simulink model "LandingGearMode"  (R2015a)
settings: Solver=FixedStepDiscrete  StartTime=0.0  StopTime=10.0  FixedStep=0.2  RelTol=1e-3
PreLoadFcn:
  | load busdata;
settings Model: RecordCoverage=on  Creator=syoon  LastModifiedBy=syoon
settings OptimizationCC: BlockReduction=off  InlineParams=on  UseDivisionForNetSlopeComputation=on  ExpressionDepthLimit=2147483647  EfficientFloat2IntCast=on  EfficientMapNaN2IntZero=off  OptimizeModelRefInitCode=on  MaxStackSize=inf
settings DebuggingCC: SignalInfNanChecking=error  SignalRangeChecking=error  ReadBeforeWriteMsg=EnableAllAsError  WriteAfterWriteMsg=EnableAllAsError  WriteAfterReadMsg=EnableAllAsError  AlgebraicLoopMsg=error  ArtificialAlgebraicLoopMsg=error  SaveWithDisabledLinksMsg=error  SaveWithParameterizedLinksMsg=error  BlockPriorityViolationMsg=error  SolverPrmCheckMsg=error  InheritedTsInSrcMsg=error  DiscreteInheritContinuousMsg=error  SigSpecEnsureSampleTimeMsg=error  CheckMatrixSingularityMsg=error  IntegerOverflowMsg=error  ParameterUnderflowMsg=error  ParameterPrecisionLossMsg=error  ParameterTunabilityLossMsg=error  UnderSpecifiedDataTypeMsg=error  UnnecessaryDatatypeConvMsg=warning  VectorMatrixConversionMsg=error  SignalLabelMismatchMsg=error  UnconnectedInputMsg=error  UnconnectedOutputMsg=error  UnconnectedLineMsg=error  SFcnCompatibilityMsg=error  BusObjectLabelMismatch=error  RootOutportRequireBusObject=error  ModelReferenceIOMsg=error  ModelReferenceIOMismatchMessage=error  UnknownTsInhSupMsg=error  ModelReferenceDataLoggingMessage=error  StateNameClashWarn=warning  StrictBusMsg=ErrorOnBusTreatedAsVector  NonBusSignalsTreatedAsBus=error  SFUnexpectedBacktrackingDiag=error  SFInvalidInputDataAccessInChartInitDiag=error  SFNoUnconditionalDefaultTransitionDiag=error  SFTransitionOutsideNaturalParentDiag=error  SFUnconditionalTransitionShadowingDiag=error  SFUndirectedBroadcastEventsDiag=error  SFTransitionActionBeforeConditionDiag=error  IntegerSaturationMsg=error
settings HardwareCC: ProdIntDivRoundTo=Zero  ProdEndianess=LittleEndian  ProdHWDeviceType=Intel->x86/Pentium  TargetBitPerLong=64  TargetBitPerPointer=64  TargetIntDivRoundTo=Zero  TargetEndianess=LittleEndian  TargetWordSize=64  TargetHWDeviceType=Intel->x86-64
settings RTWCC: SystemTargetFile=ert.tlc  TemplateMakefile=ert_default_tmf  Description=Embedded Coder  GenerateReport=on  IncludeHyperlinkInReport=on  LaunchReport=on  PortableWordSizes=on  CodeExecutionProfiling=on  CodeProfilingInstrumentation=on  GenerateTraceInfo=on  GenerateTraceReport=on  GenerateTraceReportSl=on  GenerateTraceReportSf=on  GenerateTraceReportEml=on  GenerateCodeMetricsReport=on
settings CodeAppCC: ForceParamTrailComments=on  IgnoreCustomStorageClasses=off  MangleLength=4  CustomSymbolStrType=$N$R$M  ReqsInCode=on
settings ERTTargetCC: UtilityFuncGeneration=Shared location  ParMdlRefBuildCompliant=on  CompOptLevelCompliant=on  ConcurrentExecutionCompliant=on  IncludeMdlTerminateFcn=off  GeneratePreprocessorConditionals=Disable all  SuppressErrorStatus=on  ERTFirstTimeCompliant=on  SupportAbsoluteTime=off  SupportNonFinite=off  SupportComplex=off  SupportContinuousTime=off  SupportVariableSizeSignals=off  ParenthesesLevel=Maximum  ModelStepFunctionPrototypeControlCompliant=on  CPPClassGenCompliant=on  GenerateSharedConstants=off  ERTCustomFileTemplate=example_file_process.tlc  PreserveExpressionOrder=on  PreserveIfCondition=on  EnableSignedLeftShifts=off
settings ConfigComp: Description=Design Verifier Custom Configuration Component  DVModelCoverageObjectives=MCDC  DVMaxTestCaseSteps=500  DVTestSuiteOptimization=CombinedObjectives (Nonlinear Extended)  DVCoverageDataFile=existingcov.cvt  DVDetectActiveLogic=on  DVSaveHarnessModel=on  DVModelReferenceHarness=on  PSVerificationSettings=PrjConfigAndMisra  PSOpenProjectManager=on  PSAutoStubLUT=off

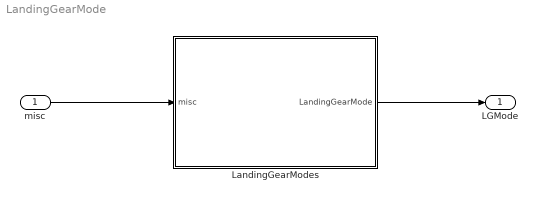
== system LandingGearMode ==
  misc : Inport  RequirementInfo={'other' '..\requirements\DisplaySystemRequirements.docx' '@Simulink_requirement_item_33' 'true' 'The state of the landing gear will be contained in a bus object: MiscData. This bus object is defined as follows:' '' } %GIDa_09af1f37_fea8_4fc2_b25f_3c32d9062372  OutDataTypeStr=Bus: MiscData  PortDimensions=1  SampleTime=0.2  BusOutputAsStruct=on
  LandingGearModes : Stateflow chart  RequirementInfo={'other' '..\requirements\DisplaySystemRequirements.docx' '@Simulink_requirement_item_35' 'true' 'The LGLeftLock and LGRightLock elements of the bus will be used to determine the output of the system: LandingGearMode.' '' } %GIDa_9a49dfa8_e211_495d_8d12_c7afe2a8f08f  TreatAsAtomicUnit=on
      settings: RTWSystemCode=Inline
  LGMode : Outport  RequirementInfo={'other' '..\requirements\DisplaySystemRequirements.docx' '@Simulink_requirement_item_34' 'true' 'The output of the system shall be an integer of type double, LandingGearMode.' '' } %GIDa_2f617b6c_313d_4ee6_8d3d_1e307f4a7039
  wires:
  LandingGearModes/1(LandingGearMode) -> LGMode/1
  misc/1 -> LandingGearModes/1(misc)

== stateflow chart LandingGearMode/LandingGearModes ==
  state LeftLock [parallel]
    settings: executionOrder=1
    state Unlocked
    state Locked
    (default) -> (junction 122)
    (junction 122) -> LeftLock.Unlocked [order 2]
    (junction 122) -> LeftLock.Locked [order 1] : [misc.LGLeftLock]
    LeftLock.Locked -> LeftLock.Unlocked : [~misc.LGLeftLock]
    LeftLock.Unlocked -> LeftLock.Locked : [misc.LGLeftLock]
  state RightLock [parallel]
    settings: executionOrder=2
    state Unlocked
    state Locked
    (default) -> (junction 136)
    (junction 136) -> RightLock.Unlocked [order 2]
    (junction 136) -> RightLock.Locked [order 1] : [misc.LGRightLock]
    RightLock.Locked -> RightLock.Unlocked : [~misc.LGRightLock]
    RightLock.Unlocked -> RightLock.Locked : [misc.LGRightLock]
  state WarningModes [parallel]
    settings: executionOrder=3
    state BothLocked
      entry:
      LandingGearMode = 1;
    state BothUnLocked
      entry:
      LandingGearMode = 3;
    state OnlyOneLocked
      entry:
      LandingGearMode = 2;
    (default) -> (junction 102)
    (junction 102) -> BothLocked [order 1] : [in(LeftLock.Locked) &&...
        | in(RightLock.Locked)]
    (junction 102) -> BothUnLocked [order 2] : [in(LeftLock.Unlocked) &&...
        | in(RightLock.Unlocked)]
    (junction 102) -> OnlyOneLocked [order 3]
    BothUnLocked -> OnlyOneLocked [order 1] : [in(LeftLock.Locked) ||...
        | in(RightLock.Locked)]
    OnlyOneLocked -> BothLocked [order 2] : [in(LeftLock.Locked) &&...
        | in(RightLock.Locked)]
    OnlyOneLocked -> BothUnLocked [order 1] : [in(LeftLock.Unlocked) &&...
        | in(RightLock.Unlocked)]
    BothLocked -> OnlyOneLocked [order 2] : [in(LeftLock.Unlocked) ||...
        | in(RightLock.Unlocked)]
    BothLocked -> BothUnLocked [order 1] : [in(LeftLock.Unlocked) &&...
        | in(RightLock.Unlocked)]
    BothUnLocked -> BothLocked [order 2] : [in(LeftLock.Locked) &&...
        | in(RightLock.Locked)]
  data: misc input Bus: MiscData; LandingGearMode output double size=1
